simulink model "test_delfttyre_cpi"  (Simulink 6.4)
settings: Solver=ode45  SolverMode=SingleTasking  StartTime=0.0  StopTime=2*pi  FixedStep=0.02  MaxStep=0.01  RelTol=1e-5  AbsTol=1e-5
libraries: simulink x2, Delft_Tyre_dtlib x1, Delft_Tyre_sm1glib x1
settings Model: Creator=hofstadrhmtvd  LastModifiedBy=hofstadrhmtvd  ExtModeTrigMode=oneshot  ExtModeArmWhenConnect=off
settings SolverCC: InitialStep=0.001
settings DataIOCC: LimitDataPoints=off  SignalLoggingName=sigsOut
settings OptimizationCC: BooleanDataType=off
settings DebuggingCC: SolverPrmCheckMsg=none  StrictBusMsg=ErrorLevel1
settings HardwareCC: TargetHWDeviceType=32-bit Generic  TargetUnknown=on  ProdEqTarget=off

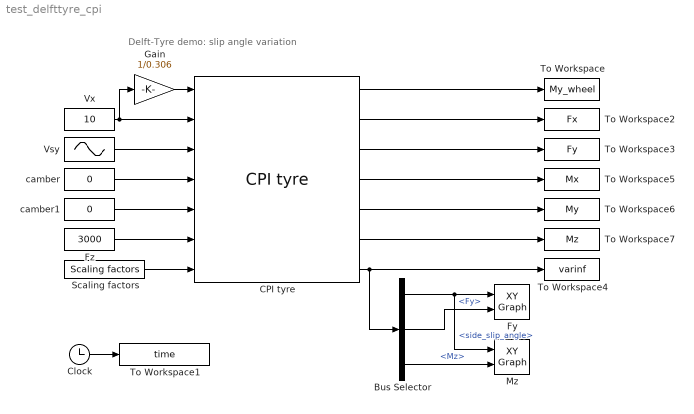
== system test_delfttyre_cpi ==
  note: Delft-Tyre demo: slip angle variation
  Bus Selector : BusSelector  OutputSignals=side_slip_angle,Fy,Mz
  CPI tyre : Delft_Tyre_dtlib/Simulink/CPI tyre  Tag=CPI tyre  SystemSampleTime=-1  idtyre=1  tpfname='TNO_car205_60R15.tir'  side_mode=(3xxx) symmetric  dyn_mode=(xx0x) steady-state  mf_mode=(xxx4) combined  use_mode=1e8  disp_debug=off
  Clock : Clock
      settings: Decimation=10
  Fy : simulink/Sinks/XY Graph  SystemSampleTime=-1  xmin=-0.2  xmax=0.2  ymin=-3500  ymax=3500  st=-1
  Fz : Constant  Value=3000  OutDataType=sfix(16)  ConRadixGroup=Use specified scaling  OutScaling=2^0  SampleTime=inf  FramePeriod=inf
  Gain : Gain  Gain=1/0.306  SaturateOnIntegerOverflow=on
  Mz : simulink/Sinks/XY Graph  SystemSampleTime=-1  xmin=-0.2  xmax=0.2  ymin=-50  ymax=50  st=-1
  Scaling factors : Delft_Tyre_sm1glib/SimMechanics 1G/Scaling factors  Tag=Scaling factors  SystemSampleTime=-1  LMUX=1  LKX=1  LMUY=1  LKY=1  LKYC=1  LTR=1  LKZC=1
  To Workspace : ToWorkspace  VariableName=My_wheel  SampleTime=-1  SaveFormat=Array
  To Workspace1 : ToWorkspace  VariableName=time  SampleTime=-1  SaveFormat=Array
  To Workspace2 : ToWorkspace  VariableName=Fx  SampleTime=-1  SaveFormat=Array
  To Workspace3 : ToWorkspace  VariableName=Fy  SampleTime=-1  SaveFormat=Array
  To Workspace4 : ToWorkspace  VariableName=varinf  SampleTime=-1  SaveFormat=Array
  To Workspace5 : ToWorkspace  VariableName=Mx  SampleTime=-1  SaveFormat=Array
  To Workspace6 : ToWorkspace  VariableName=My  SampleTime=-1  SaveFormat=Array
  To Workspace7 : ToWorkspace  VariableName=Mz  SampleTime=-1  SaveFormat=Array
  Vsy : Sin  Amplitude=2  SampleTime=0
  Vx : Constant  Value=10  OutDataType=sfix(16)  ConRadixGroup=Use specified scaling  OutScaling=2^0  SampleTime=inf  FramePeriod=inf
  camber : Constant  Value=0  OutDataType=sfix(16)  ConRadixGroup=Use specified scaling  OutScaling=2^0  SampleTime=inf  FramePeriod=inf
  camber1 : Constant  Value=0  OutDataType=sfix(16)  ConRadixGroup=Use specified scaling  OutScaling=2^0  SampleTime=inf  FramePeriod=inf
  wires:
  Clock/1 -> To Workspace1/1
  Scaling factors/1 -> CPI tyre/7
  Vsy/1 -> CPI tyre/3
  camber/1 -> CPI tyre/4
  Fz/1 -> CPI tyre/6
  CPI tyre/1 -> To Workspace/1
  CPI tyre/2 -> To Workspace2/1
  CPI tyre/3 -> To Workspace3/1
  CPI tyre/4 -> To Workspace5/1
  CPI tyre/6 -> To Workspace7/1
  CPI tyre/5 -> To Workspace6/1
  Vx/1 -> Gain/1, CPI tyre/2
  CPI tyre/7 -> To Workspace4/1, Bus Selector/1
  Bus Selector/1 -> Fy/1, Mz/1  "<side_slip_angle>"
  Bus Selector/2 -> Fy/2  "<Fy>"
  Bus Selector/3 -> Mz/2  "<Mz>"
  Gain/1 -> CPI tyre/1
  camber1/1 -> CPI tyre/5
